simulink model "FixedWing_Dynamic_Model_SIL_simulink_PX4_H200"  (R2023a)
settings: Solver=ode4  StartTime=0.0  StopTime=130  FixedStep=0.004  RelTol=1e-3
model workspace (MAT data in the model file):
  sample_time = 0.004
values from neighbouring files (symbols this model uses):
  ref_height = 171    [InitSimulinkPlantVars.m]
  ref_lat = 39.49738807491014    (= 39.4973880749)    [InitSimulinkPlantVars.m]
  ref_lon = -0.6268122488722822    (= -0.626812248872)    [InitSimulinkPlantVars.m]
undefined symbols (not defined in the file or in its folder): DiscIntNeverNeededParam, Earth, env, frecuency, g, LC, mission, nwap, pitch_D, pitch_ff, pitch_I, pitch_P, poswp, roll_D, roll_ff, roll_I, roll_P, tc_pitch, tc_roll, TEBCL, TECL, TECS, uavData, V_cruise, WGS84, yaw_D, yaw_ff, yaw_I, yaw_P
libraries: aerolibactuator x5, aerolibasang x4, slpidlib x3, uavalgslib x2, aerolibatmos2 x2, shared6dof x1, aerolibtransform2 x1, simulink_extras x1
(part 2 of 3)

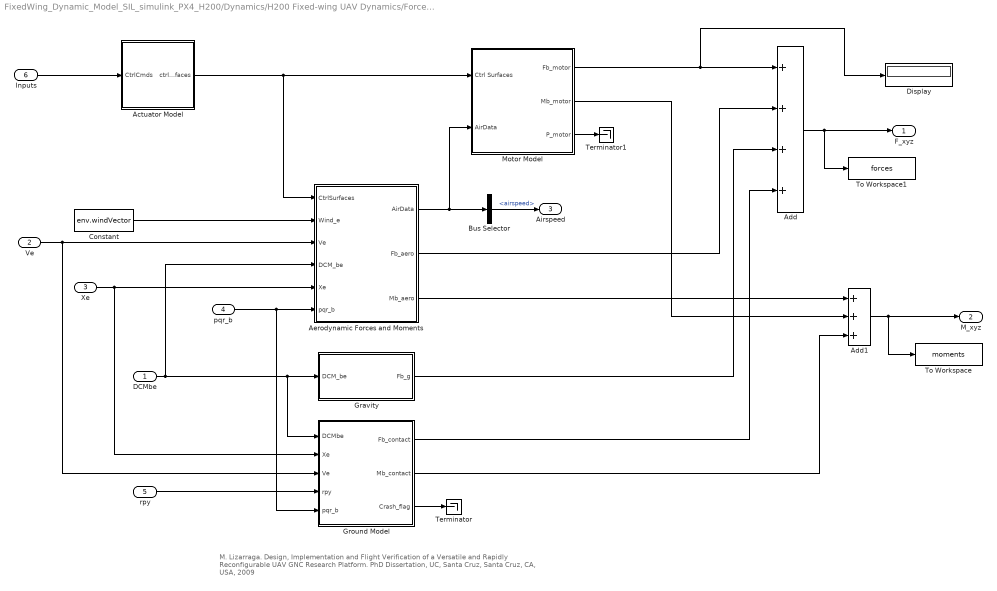
== system FixedWing_Dynamic_Model_SIL_simulink_PX4_H200/Dynamics/H200 Fixed-wing UAV Dynamics/Force and Moment Calculation ==
  note: M. Lizarraga. Design, Implementation and Flight Verification of a Versatile and Rapidly Reconfigurable UAV GNC Research Platform. PhD Dissertation, UC, Santa Cruz, Santa Cruz, CA, USA, 2009
  DCMbe : Inport
  Ve : Inport  Port=2
  Xe : Inport  Port=3
  pqr_b : Inport  Port=4
  rpy : Inport  Port=5
  Inputs : Inport  Port=6
  Actuator Model : Subsystem
  Add : Sum  Inputs=4
  Add1 : Sum  Inputs=+++
  Aerodynamic Forces and Moments : Subsystem
  Bus Selector : BusSelector  OutputSignals=airspeed
  Constant : Constant  Value=env.windVector
  Display : Display
  Gravity : Subsystem
  Ground Model : Subsystem
  Motor Model : Subsystem
  Terminator : Terminator
  Terminator1 : Terminator
  To Workspace : ToWorkspace  VariableName=moments  SaveFormat=Timeseries  SampleTime=-1
  To Workspace1 : ToWorkspace  VariableName=forces  SaveFormat=Timeseries  SampleTime=-1
  F_xyz : Outport
  M_xyz : Outport  Port=2
  Airspeed : Outport  Port=3
  wires:
  Add/1 -> To Workspace1/1, F_xyz/1
  DCMbe/1 -> Ground Model/1(DCMbe), Gravity/1(DCM_be), Aerodynamic Forces and Moments/4(DCM_be)
  pqr_b/1 -> Aerodynamic Forces and Moments/6(pqr_b), Ground Model/5(pqr_b)
  Actuator Model/1(ctrlSurfaces) -> Aerodynamic Forces and Moments/1(CtrlSurfaces), Motor Model/1(Ctrl Surfaces)
  Aerodynamic Forces and Moments/1(AirData) -> Motor Model/2(AirData), Bus Selector/1
  Ground Model/1(Fb_contact) -> Add/4
  Gravity/1(Fb_g) -> Add/3
  Motor Model/1(Fb_motor) -> Display/1, Add/1
  Ve/1 -> Aerodynamic Forces and Moments/3(Ve), Ground Model/3(Ve)
  Ground Model/3(Crash_flag) -> Terminator/1
  Aerodynamic Forces and Moments/2(Fb_aero) -> Add/2
  Aerodynamic Forces and Moments/3(Mb_aero) -> Add1/1
  Xe/1 -> Aerodynamic Forces and Moments/5(Xe), Ground Model/2(Xe)
  Constant/1 -> Aerodynamic Forces and Moments/2(Wind_e)
  Inputs/1 -> Actuator Model/1(CtrlCmds)
  Bus Selector/1 -> Airspeed/1  "<airspeed>"
  rpy/1 -> Ground Model/4(rpy)
  Add1/1 -> M_xyz/1, To Workspace/1
  Ground Model/2(Mb_contact) -> Add1/3
  Motor Model/2(Mb_motor) -> Add1/2
  Motor Model/3(P_motor) -> Terminator1/1

== system FixedWing_Dynamic_Model_SIL_simulink_PX4_H200/Controllers/Total Energy control system/Total energy balance control loop/ B SP dot ==
  h : Inport  SampleTime=frecuency
  V_TAS : Inport  Port=2  SampleTime=frecuency
  V_TAS_sp : Inport  Port=3  SampleTime=frecuency
  h_sp : Inport  Port=4  SampleTime=frecuency
  h_rate_sp : Inport  Port=5  SampleTime=frecuency
  weight_ske : Inport  Port=6  SampleTime=frecuency
  weight_spe : Inport  Port=7  SampleTime=frecuency
  Add : Sum  Inputs=-+
  Add1 : Sum  Inputs=-+
  Add2 : Sum  Inputs=-+
  Add3 : Sum
  Constant : Constant  Value=TECL.V_error_gain  SampleTime=frecuency
  Constant1 : Constant  Value=TECL.h_error_gain  SampleTime=frecuency
  Constant2 : Constant  Value=TECL.h_ff_gain  SampleTime=frecuency
  Constant3 : Constant  Value=g  SampleTime=frecuency
  Product1 : Product
  Product2 : Product  Inputs=3
  Product3 : Product
  Product4 : Product
  Product5 : Product  Inputs=3
  Bdot SP : Outport  SampleTime=frecuency
  wires:
  V_TAS_sp/1 -> Add1/2
  Product1/1 -> Product2/2
  Product2/1 -> Add/1  "kinetic"
  h_sp/1 -> Add2/2
  h/1 -> Add2/1
  Add2/1 -> Product4/2
  Constant1/1 -> Product4/1
  Product4/1 -> Add3/1
  Constant2/1 -> Product3/1
  Product3/1 -> Add3/2
  Add3/1 -> Product5/2
  Constant3/1 -> Product5/1
  Product5/1 -> Add/2  "potential"
  Add/1 -> Bdot SP/1
  h_rate_sp/1 -> Product3/2
  weight_ske/1 -> Product2/3
  weight_spe/1 -> Product5/3
  V_TAS/1 -> Add1/1, Product2/1
  Add1/1 -> Product1/1
  Constant/1 -> Product1/2

== system FixedWing_Dynamic_Model_SIL_simulink_PX4_H200/Controllers/Total Energy control system/Total energy balance control loop/Bdot ==
  V_TAS : Inport  SampleTime=frecuency
  V_rate : Inport  Port=2  SampleTime=frecuency
  h_rate : Inport  Port=3  SampleTime=frecuency
  weight_ske : Inport  Port=4  SampleTime=frecuency
  weight_spe : Inport  Port=5  SampleTime=frecuency
  Add : Sum  Inputs=-+
  Constant : Constant  Value=g  SampleTime=frecuency
  Product : Product  Inputs=3
  Product1 : Product  Inputs=3
  Bdot : Outport  SampleTime=frecuency
  wires:
  V_rate/1 -> Product/2
  Constant/1 -> Product1/3
  h_rate/1 -> Product1/2
  Product/1 -> Add/1  "kinetic"
  Product1/1 -> Add/2  "potential"
  Add/1 -> Bdot/1
  weight_ske/1 -> Product/3
  weight_spe/1 -> Product1/1
  V_TAS/1 -> Product/1

== system FixedWing_Dynamic_Model_SIL_simulink_PX4_H200/Controllers/Total Energy control system/Total energy balance control loop/pitchdotsp - pitchFF ==
  Bdot SP : Inport  SampleTime=frecuency
  Gain : Gain  Gain=TEBCL.rate_ff
  pitch_FF : Outport  SampleTime=frecuency
  wires:
  Bdot SP/1 -> Gain/1
  Gain/1 -> pitch_FF/1

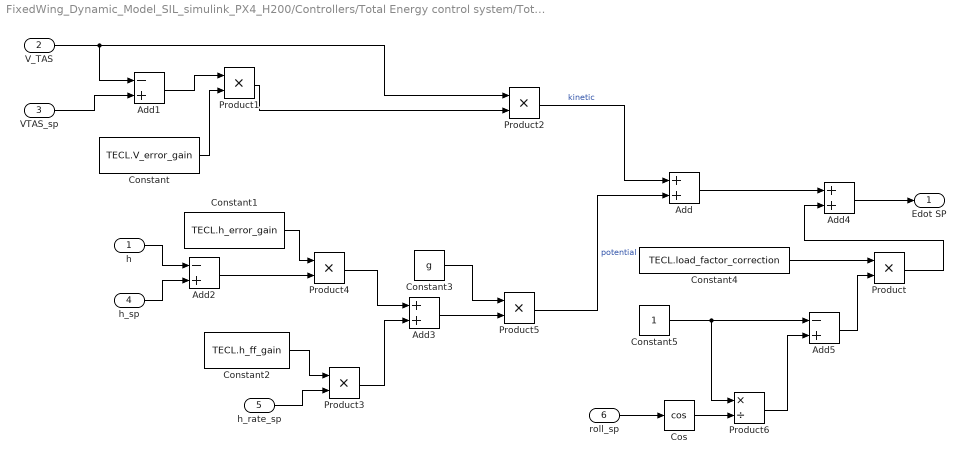
== system FixedWing_Dynamic_Model_SIL_simulink_PX4_H200/Controllers/Total Energy control system/Total energy control loop/E SP dot ==
  h : Inport  SampleTime=frecuency
  V_TAS : Inport  Port=2  SampleTime=frecuency
  VTAS_sp : Inport  Port=3  SampleTime=frecuency
  h_sp : Inport  Port=4  SampleTime=frecuency
  h_rate_sp : Inport  Port=5  SampleTime=frecuency
  roll_sp : Inport  Port=6  SampleTime=frecuency
  Add : Sum
  Add1 : Sum  Inputs=-+
  Add2 : Sum  Inputs=-+
  Add3 : Sum
  Add4 : Sum
  Add5 : Sum  Inputs=-+
  Constant : Constant  Value=TECL.V_error_gain  SampleTime=frecuency
  Constant1 : Constant  Value=TECL.h_error_gain  SampleTime=frecuency
  Constant2 : Constant  Value=TECL.h_ff_gain  SampleTime=frecuency
  Constant3 : Constant  Value=g
  Constant4 : Constant  Value=TECL.load_factor_correction  SampleTime=frecuency
  Constant5 : Constant
  Cos : Trigonometry  Operator=cos
  Product{,1..5} (6 alike) : Product
  Product6 : Product  Inputs=*/
  Edot SP : Outport  SampleTime=frecuency
  wires:
  VTAS_sp/1 -> Add1/2
  Product2/1 -> Add/1  "kinetic"
  h_sp/1 -> Add2/2
  h/1 -> Add2/1
  Add2/1 -> Product4/2
  Constant1/1 -> Product4/1
  Product4/1 -> Add3/1
  Constant2/1 -> Product3/1
  Product3/1 -> Add3/2
  Add3/1 -> Product5/2
  Constant3/1 -> Product5/1
  Product5/1 -> Add/2  "potential"
  h_rate_sp/1 -> Product3/2
  Add/1 -> Add4/1
  Add4/1 -> Edot SP/1
  Constant4/1 -> Product/1
  Product/1 -> Add4/2
  Constant5/1 -> Add5/1, Product6/1
  Add5/1 -> Product/2
  roll_sp/1 -> Cos/1
  Cos/1 -> Product6/2
  Product6/1 -> Add5/2
  Constant/1 -> Product1/2
  Add1/1 -> Product1/1
  Product1/1 -> Product2/2
  V_TAS/1 -> Product2/1, Add1/1

== system FixedWing_Dynamic_Model_SIL_simulink_PX4_H200/Controllers/Total Energy control system/Total energy control loop/Edot ==
  V_TAS : Inport  SampleTime=frecuency
  V_rate : Inport  Port=2  SampleTime=frecuency
  h_rate : Inport  Port=3  SampleTime=frecuency
  Add : Sum
  Constant : Constant  Value=g  SampleTime=frecuency
  Product : Product
  Product1 : Product
  Edot : Outport  SampleTime=frecuency
  wires:
  V_TAS/1 -> Product/1
  V_rate/1 -> Product/2
  Constant/1 -> Product1/2
  h_rate/1 -> Product1/1
  Product/1 -> Add/1  "kinetic"
  Product1/1 -> Add/2  "potential"
  Add/1 -> Edot/1

== system FixedWing_Dynamic_Model_SIL_simulink_PX4_H200/Controllers/Total Energy control system/Total energy control loop/Subsystem ==
  ratio_undersped : Inport  SampleTime=frecuency
  T_sp : Inport  Port=2  SampleTime=frecuency
  Tmax : Inport  Port=3  SampleTime=frecuency
  Add : Sum  Inputs=+-
  Add1 : Sum
  Constant : Constant  SampleTime=frecuency
  Product : Product
  Product1 : Product
  throttle_setpoint : Outport  SampleTime=frecuency
  wires:
  ratio_undersped/1 -> Product/1, Add/2
  Tmax/1 -> Product/2
  Constant/1 -> Add/1
  T_sp/1 -> Product1/1
  Add/1 -> Product1/2
  Product1/1 -> Add1/1
  Product/1 -> Add1/2
  Add1/1 -> throttle_setpoint/1

== system FixedWing_Dynamic_Model_SIL_simulink_PX4_H200/Controllers/Total Energy control system/Total energy control loop/Subsystem1 ==
  throttle_integ_input : Inport  SampleTime=frecuency
  ste_rate_to_throttle : Inport  Port=2  SampleTime=frecuency
  ratio_undersped : Inport  Port=3  SampleTime=frecuency
  Add : Sum  Inputs=-+
  Constant : Constant  SampleTime=frecuency
  Product : Product  Inputs=3
  throttle_integ : Outport  SampleTime=frecuency
  wires:
  ratio_undersped/1 -> Add/1
  Constant/1 -> Add/2
  throttle_integ_input/1 -> Product/1
  ste_rate_to_throttle/1 -> Product/2
  Add/1 -> Product/3
  Product/1 -> throttle_integ/1

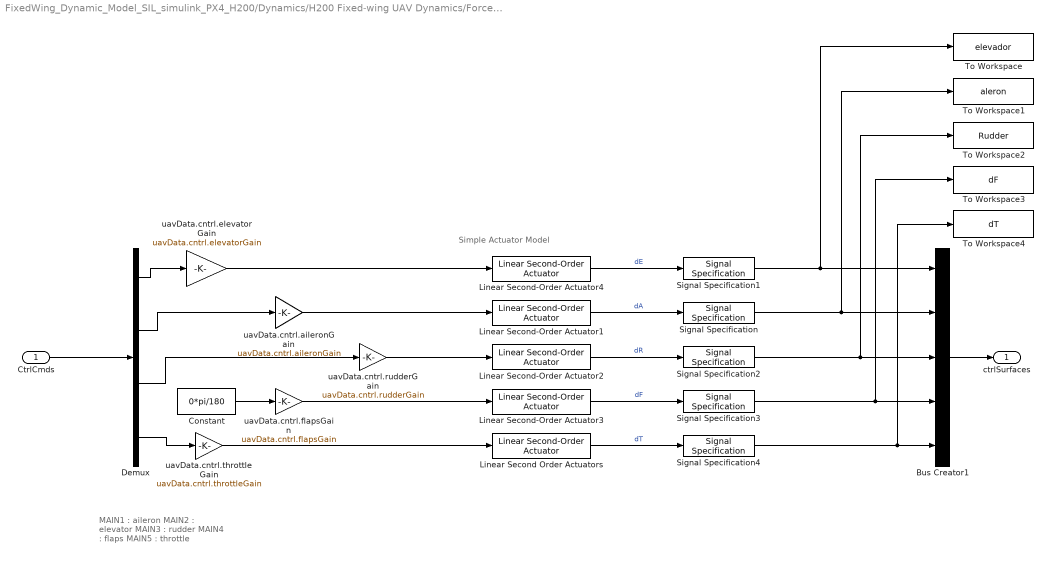
== system FixedWing_Dynamic_Model_SIL_simulink_PX4_H200/Dynamics/H200 Fixed-wing UAV Dynamics/Force and Moment Calculation/Actuator Model ==
  note: Simple Actuator Model
  note: MAIN1 : aileron
      | MAIN2 : elevator
      | MAIN3 : rudder
      | MAIN4 : flaps
      | MAIN5 : throttle
  CtrlCmds : Inport
  Bus Creator1 : BusCreator  Inputs=5
  Constant : Constant  Value=0*pi/180
  Demux : Demux
  Linear Second Order Actuators : aerolibactuator/Linear Second-Order Actuator  wn_fin=uavData.cntrl.naturalFreq  z_fin=uavData.cntrl.dampingRatio  fin_act_0=uavData.cntrl.initPos  fin_act_vel=uavData.cntrl.initVel
      settings: AttributesFormatString=|
      | Nat Freq => %<wn_fin>
      | Damping => %<z_fin>
  Linear Second-Order Actuator{1..4} (4 alike) : aerolibactuator/Linear Second-Order Actuator  wn_fin=uavData.cntrl.naturalFreq  z_fin=uavData.cntrl.dampingRatio  fin_act_0=uavData.cntrl.initPos  fin_act_vel=uavData.cntrl.initVel
  Signal Specification{,1..3} (4 alike) : SignalSpecification  Unit=rad
  Signal Specification4 : SignalSpecification  Unit=%
  To Workspace : ToWorkspace  VariableName=elevador  SaveFormat=Timeseries  SampleTime=-1
  To Workspace1 : ToWorkspace  VariableName=aleron  SaveFormat=Timeseries  SampleTime=-1
  To Workspace2 : ToWorkspace  VariableName=Rudder  SaveFormat=Timeseries  SampleTime=-1
  To Workspace3 : ToWorkspace  VariableName=dF  SaveFormat=Timeseries  SampleTime=-1
  To Workspace4 : ToWorkspace  VariableName=dT  SaveFormat=Timeseries  SampleTime=-1
  uavData.cntrl.aileronGain : Gain  Gain=uavData.cntrl.aileronGain
  uavData.cntrl.elevatorGain : Gain  Gain=uavData.cntrl.elevatorGain
  uavData.cntrl.flapsGain : Gain  Gain=uavData.cntrl.flapsGain
  uavData.cntrl.rudderGain : Gain  Gain=uavData.cntrl.rudderGain
  uavData.cntrl.throttleGain : Gain  Gain=uavData.cntrl.throttleGain
  ctrlSurfaces : Outport  VectorParamsAs1DForOutWhenUnconnected=off
  wires:
  uavData.cntrl.throttleGain/1 -> Linear Second Order Actuators/1
  Bus Creator1/1 -> ctrlSurfaces/1
  Linear Second-Order Actuator4/1 -> Signal Specification1/1  "dE"
  Linear Second-Order Actuator1/1 -> Signal Specification/1  "dA"
  Linear Second-Order Actuator2/1 -> Signal Specification2/1  "dR"
  Linear Second-Order Actuator3/1 -> Signal Specification3/1  "dF"
  Linear Second Order Actuators/1 -> Signal Specification4/1  "dT"
  CtrlCmds/1 -> Demux/1
  Signal Specification1/1 -> To Workspace/1, Bus Creator1/1
  Signal Specification/1 -> To Workspace1/1, Bus Creator1/2
  Signal Specification2/1 -> To Workspace2/1, Bus Creator1/3
  Signal Specification3/1 -> To Workspace3/1, Bus Creator1/4
  Signal Specification4/1 -> Bus Creator1/5, To Workspace4/1
  Demux/3 -> uavData.cntrl.rudderGain/1
  Demux/1 -> uavData.cntrl.elevatorGain/1
  Demux/2 -> uavData.cntrl.aileronGain/1
  uavData.cntrl.elevatorGain/1 -> Linear Second-Order Actuator4/1
  uavData.cntrl.rudderGain/1 -> Linear Second-Order Actuator2/1
  uavData.cntrl.aileronGain/1 -> Linear Second-Order Actuator1/1
  uavData.cntrl.flapsGain/1 -> Linear Second-Order Actuator3/1
  Demux/4 -> uavData.cntrl.throttleGain/1
  Constant/1 -> uavData.cntrl.flapsGain/1

== system FixedWing_Dynamic_Model_SIL_simulink_PX4_H200/Dynamics/H200 Fixed-wing UAV Dynamics/Force and Moment Calculation/Aerodynamic Forces and Moments ==
  CtrlSurfaces : Inport
  Wind_e : Inport  Port=2
  Ve : Inport  Port=3
  DCM_be : Inport  Port=4
  Xe : Inport  Port=5
  pqr_b : Inport  Port=6
  Compute Air Data : Subsystem  TreatAsAtomicUnit=on  VariantControl=use_aerospace_blocks == 1
  Compute Body Frame Forces and Moments : Subsystem
  Compute Rho : Subsystem
  Rotate Vw : Subsystem
  Vair : Sum  Inputs=+-  InputSameDT=on  SaturateOnIntegerOverflow=on  OutDataTypeStr=Inherit: Same as first input
  AirData : Outport  VectorParamsAs1DForOutWhenUnconnected=off
  Fb_aero : Outport  Port=2
  Mb_aero : Outport  Port=3
  wires:
  Ve/1 -> Vair/1
  Compute Body Frame Forces and Moments/1(F_b) -> Fb_aero/1
  Wind_e/1 -> Vair/2
  CtrlSurfaces/1 -> Compute Body Frame Forces and Moments/2(CtrlSurfaces)
  Compute Air Data/1(AirData) -> Compute Body Frame Forces and Moments/1(AirData), AirData/1
  Compute Body Frame Forces and Moments/2(M_b) -> Mb_aero/1
  Rotate Vw/1(Vb) -> Compute Air Data/1(Vb)
  Compute Rho/1(Rho) -> Compute Air Data/2(Rho)
  Vair/1 -> Rotate Vw/1(Vw)
  pqr_b/1 -> Compute Body Frame Forces and Moments/3(p,q,r)
  DCM_be/1 -> Rotate Vw/2(DCM_be)
  Xe/1 -> Compute Rho/1(Xe)

== system FixedWing_Dynamic_Model_SIL_simulink_PX4_H200/Dynamics/H200 Fixed-wing UAV Dynamics/Force and Moment Calculation/Gravity ==
  DCM_be : Inport
  Constant : Constant  Value=[0 0 env.ISA_g]'
  Gain : Gain  Gain=uavData.geometry.m
  Matrix Multiply : Product  Multiplication=Matrix(*)
  Fb_g : Outport
  wires:
  Matrix Multiply/1 -> Gain/1
  Constant/1 -> Matrix Multiply/2
  DCM_be/1 -> Matrix Multiply/1
  Gain/1 -> Fb_g/1

== system FixedWing_Dynamic_Model_SIL_simulink_PX4_H200/Dynamics/H200 Fixed-wing UAV Dynamics/Force and Moment Calculation/Ground Model ==
  note: Body is assumed to be a rigid point mass on ground for contact force calculations.
      |
      | Normal force is modelled as a spring mass damper.
      |
      | Friction is modelled using Soft Coulomb model.
  DCMbe : Inport
  Xe : Inport  Port=2
  Ve : Inport  Port=3
  rpy : Inport  Port=4
  pqr_b : Inport  Port=5
  Constant : Constant  Value=[0 0 0]
  Crash Detector : Subsystem
  Friction Force : Subsystem
  Matrix Multiply : Product  Multiplication=Matrix(*)
  Mux1 : Mux  Inputs=2
  Normal Force : Subsystem
  Selector : Selector  InputPortWidth=3  IndexOptions=Index vector (dialog)  Indices=[3]  OutputSizes=1
  Selector1 : Selector  InputPortWidth=3  IndexOptions=Index vector (dialog)  Indices=[3]  OutputSizes=1
  Selector2 : Selector  InputPortWidth=3  IndexOptions=Index vector (dialog)  Indices=[1,2]  OutputSizes=1
  Terminator : Terminator
  Terminator1 : Terminator
  Unary Minus1 : UnaryMinus
  Fb_contact : Outport
  Mb_contact : Outport  Port=2
  Crash_flag : Outport  Port=3
  wires:
  Crash Detector/1(crashFlag) -> Crash_flag/1
  Xe/1 -> Selector/1
  Ve/1 -> Selector2/1, Selector1/1
  Selector1/1 -> Normal Force/1(Vz)
  Selector/1 -> Normal Force/2(Z)
  DCMbe/1 -> Matrix Multiply/1
  Matrix Multiply/1 -> Fb_contact/1
  Normal Force/1(Normal) -> Friction Force/2(Fn), Unary Minus1/1
  Mux1/1 -> Matrix Multiply/2, Crash Detector/1(F)
  Unary Minus1/1 -> Mux1/2
  Selector2/1 -> Friction Force/1(V)
  Friction Force/1(Friction) -> Mux1/1
  pqr_b/1 -> Terminator/1
  rpy/1 -> Terminator1/1
  Constant/1 -> Mb_contact/1

== system FixedWing_Dynamic_Model_SIL_simulink_PX4_H200/Dynamics/H200 Fixed-wing UAV Dynamics/Force and Moment Calculation/Motor Model ==
  Ctrl Surfaces : Inport
  AirData : Inport  Port=2
  Bus Selector : BusSelector  OutputSignals=dT
  Constant2 : Constant  Value=uavData.geometry.LProp
  Engine Model : Subsystem
  Gain1 : Gain  Gain=-1
  Product1 : Product  Inputs=**
  Fb_motor : Outport  VectorParamsAs1DForOutWhenUnconnected=off
  Mb_motor : Outport  Port=2  VectorParamsAs1DForOutWhenUnconnected=off
  P_motor : Outport  Port=3  VectorParamsAs1DForOutWhenUnconnected=off
  wires:
  Ctrl Surfaces/1 -> Bus Selector/1
  Bus Selector/1 -> Engine Model/1(dt)  "<dT>"
  Engine Model/1(Thrust_b) -> Fb_motor/1, Product1/1
  Constant2/1 -> Product1/2
  Product1/1 -> Gain1/1
  Gain1/1 -> Mb_motor/1
  AirData/1 -> Engine Model/2(AirData)
  Engine Model/2(Power) -> P_motor/1

== system FixedWing_Dynamic_Model_SIL_simulink_PX4_H200/Dynamics/H200 Fixed-wing UAV Dynamics/Force and Moment Calculation/Aerodynamic Forces and Moments/Compute Air Data ==
  Vb : Inport  PortDimensions=3
  Rho : Inport  Port=2
  Bus Creator : BusCreator  Inputs=4
  Demux : Demux  Outputs=3
  Dynamic Pressure : aerolibasang/Dynamic Pressure
  Subsystem : Subsystem
  AirData : Outport  VectorParamsAs1DForOutWhenUnconnected=off
  wires:
  Bus Creator/1 -> AirData/1
  Rho/1 -> Dynamic Pressure/2
  Dynamic Pressure/1 -> Bus Creator/4  "q"
  Vb/1 -> Subsystem/1(Vb), Dynamic Pressure/1
  Subsystem/1(airData) -> Demux/1
  Demux/1 -> Bus Creator/1  "alpha"
  Demux/2 -> Bus Creator/2  "beta"
  Demux/3 -> Bus Creator/3  "airspeed"

== system FixedWing_Dynamic_Model_SIL_simulink_PX4_H200/Dynamics/H200 Fixed-wing UAV Dynamics/Force and Moment Calculation/Aerodynamic Forces and Moments/Compute Body Frame Forces and Moments ==
  AirData : Inport
  CtrlSurfaces : Inport  Port=2
  p,q,r : Inport  Port=3
  Bus Selector : BusSelector  OutputSignals=alpha,beta
  Mux : Mux  Inputs=2
  Rotate FM to body frame : Subsystem
  Wind frame F& M : Subsystem
  F_b : Outport  Unit=kg*m/s^2  VectorParamsAs1DForOutWhenUnconnected=off
  M_b : Outport  Port=2  Unit=N*m  VectorParamsAs1DForOutWhenUnconnected=off
  wires:
  Mux/1 -> Rotate FM to body frame/2(alpha_beta)
  Bus Selector/2 -> Mux/2  "<beta>"
  Bus Selector/1 -> Mux/1  "<alpha>"
  Wind frame F& M/1(FM_w) -> Rotate FM to body frame/1(FM_w)  "FM_W"
  p,q,r/1 -> Wind frame F& M/3(p,q,r)
  Rotate FM to body frame/2(M_b) -> M_b/1
  Rotate FM to body frame/1(F_b) -> F_b/1
  CtrlSurfaces/1 -> Wind frame F& M/2(CtrlSurfaces)
  AirData/1 -> Wind frame F& M/1(Airdata), Bus Selector/1

== system FixedWing_Dynamic_Model_SIL_simulink_PX4_H200/Dynamics/H200 Fixed-wing UAV Dynamics/Force and Moment Calculation/Aerodynamic Forces and Moments/Compute Rho ==
  Xe : Inport
  Gain : Gain  Gain=-1
      settings: AttributesFormatString=Z to Alt
  Get Z : Selector  InputPortWidth=3  IndexOptions=Index vector (dialog)  Indices=[3]  OutputSizes=[(-2)]
  ISA Atmosphere Model1 : aerolibatmos2/ISA Atmosphere Model  custom=on  g=env.ISA_g  gamma=1.4  R=env.ISA_R  L=env.ISA_lapse  h_trop=11000  h_strat=20000  rho0=env.ISA_rho0  P0=env.ISA_P0  T0=env.ISA_T0  h0=0
  Terminator : Terminator
  Terminator1 : Terminator
  Terminator2 : Terminator
  Transfer Fcn : TransferFcn  Denominator=[.01 1]
  Rho : Outport  VectorParamsAs1DForOutWhenUnconnected=off
  wires:
  ISA Atmosphere Model1/2 -> Terminator1/1
  ISA Atmosphere Model1/1 -> Terminator/1  "OAT"
  Gain/1 -> ISA Atmosphere Model1/1
  Get Z/1 -> Transfer Fcn/1
  Transfer Fcn/1 -> Gain/1
  ISA Atmosphere Model1/3 -> Terminator2/1  "static"
  Xe/1 -> Get Z/1
  ISA Atmosphere Model1/4 -> Rho/1

== system FixedWing_Dynamic_Model_SIL_simulink_PX4_H200/Dynamics/H200 Fixed-wing UAV Dynamics/Force and Moment Calculation/Aerodynamic Forces and Moments/Rotate Vw ==
  Vw : Inport
  DCM_be : Inport  Port=2
  RL2B * Vw : Product  Multiplication=Matrix(*)  InputSameDT=on  SaturateOnIntegerOverflow=on  OutDataTypeStr=Inherit: Same as first input
  Vb : Outport  Unit=m/s  VectorParamsAs1DForOutWhenUnconnected=off
  wires:
  RL2B * Vw/1 -> Vb/1
  Vw/1 -> RL2B * Vw/2
  DCM_be/1 -> RL2B * Vw/1

== system FixedWing_Dynamic_Model_SIL_simulink_PX4_H200/Dynamics/H200 Fixed-wing UAV Dynamics/Force and Moment Calculation/Ground Model/Crash Detector ==
  F : Inport
  Constant : Constant  Value=true
  Constant1 : Constant  Value=false
  Gain : Gain  Gain=1/(env.ISA_g*uavData.geometry.m)
  Switch : Switch  Criteria=u2 > Threshold  Threshold=uavData.contact.gLimit  SaturateOnIntegerOverflow=off  InputSameDT=off
  norm1 : Subsystem
  crashFlag : Outport
  wires:
  F/1 -> norm1/1(F)
  norm1/1(Out1) -> Gain/1
  Switch/1 -> crashFlag/1
  Constant/1 -> Switch/1
  Constant1/1 -> Switch/3
  Gain/1 -> Switch/2

== system FixedWing_Dynamic_Model_SIL_simulink_PX4_H200/Dynamics/H200 Fixed-wing UAV Dynamics/Force and Moment Calculation/Ground Model/Friction Force ==
  V : Inport
  Fn : Inport  Port=2
  Product : Product
  Soft Coulomb Friction : Subsystem
  Unary Minus : UnaryMinus
  Friction : Outport
  wires:
  Fn/1 -> Product/2
  Soft Coulomb Friction/1(Out1) -> Product/1
  Product/1 -> Unary Minus/1
  Unary Minus/1 -> Friction/1
  V/1 -> Soft Coulomb Friction/1(V)

== system FixedWing_Dynamic_Model_SIL_simulink_PX4_H200/Dynamics/H200 Fixed-wing UAV Dynamics/Force and Moment Calculation/Ground Model/Normal Force ==
  Vz : Inport
  Z : Inport  Port=2
  Add : Sum
  Constant : Constant  Value=0
  Damper : Gain  Gain=-uavData.contact.damper
  Saturation : Saturate  UpperLimit=inf  LowerLimit=0
  Spring Kp : Gain  Gain=-uavData.contact.spring
  Switch : Switch  Criteria=u2 > Threshold  SaturateOnIntegerOverflow=off  InputSameDT=off
  Unary Minus : UnaryMinus
  Unary Minus1 : UnaryMinus
  Normal : Outport
  wires:
  Constant/1 -> Switch/1
  Z/1 -> Unary Minus/1
  Switch/1 -> Saturation/1
  Damper/1 -> Add/2
  Add/1 -> Switch/3
  Spring Kp/1 -> Add/1
  Vz/1 -> Unary Minus1/1
  Saturation/1 -> Normal/1
  Unary Minus/1 -> Spring Kp/1, Switch/2
  Unary Minus1/1 -> Damper/1

== system FixedWing_Dynamic_Model_SIL_simulink_PX4_H200/Dynamics/H200 Fixed-wing UAV Dynamics/Force and Moment Calculation/Motor Model/Engine Model ==
  dt : Inport
  AirData : Inport  Port=2
  Constant4 : Constant  Value=0
      settings: AttributesFormatString=%<Value>
  Mux1 : Mux  Inputs=3
  Power Model : Subsystem
  Thurst Model : Subsystem
  To Workspace1 : ToWorkspace  VariableName=thrustMotor  SaveFormat=Timeseries  SampleTime=-1
  To Workspace2 : ToWorkspace  VariableName=powerMotor  SaveFormat=Timeseries  SampleTime=-1
  Thrust_b : Outport  Unit=kg*m/s^2  VectorParamsAs1DForOutWhenUnconnected=off
  Power : Outport  Port=2  Unit=kg*m/s^2  VectorParamsAs1DForOutWhenUnconnected=off
  wires:
  Constant4/1 -> Mux1/2, Mux1/3
  Mux1/1 -> Thrust_b/1
  dt/1 -> Power Model/1(dt), Thurst Model/1(dt)
  Thurst Model/1(T_Total) -> Mux1/1, To Workspace1/1
  AirData/1 -> Thurst Model/2(AirData), Power Model/2(AirData)
  Power Model/1(P_Total) -> To Workspace2/1, Power/1

== system FixedWing_Dynamic_Model_SIL_simulink_PX4_H200/Dynamics/H200 Fixed-wing UAV Dynamics/Force and Moment Calculation/Aerodynamic Forces and Moments/Compute Air Data/Subsystem ==
  note: Avoid singularity at low speeds
  Vb : Inport
  "Incidence, Sideslip, & Airspeed" : aerolibasang/Incidence, Sideslip, & Airspeed
  Mux : Mux  Inputs=3
  Mux1 : Mux  Inputs=3
  Switch : Switch  Criteria=u2 > Threshold  Threshold=0.1  SaturateOnIntegerOverflow=off  InputSameDT=off
  alpha : Constant  Value=0
  beta : Constant  Value=0
  norm : Subsystem
  airData : Outport
  wires:
  "Incidence, Sideslip, & Airspeed"/1 -> Mux/1  "alpha"
  "Incidence, Sideslip, & Airspeed"/3 -> Mux/3  "airspeed"
  Vb/1 -> norm/1(In1), "Incidence, Sideslip, & Airspeed"/1
  norm/1(Out1) -> Switch/2, Mux1/3
  "Incidence, Sideslip, & Airspeed"/2 -> Mux/2  "beta"
  Switch/1 -> airData/1
  Mux/1 -> Switch/1
  alpha/1 -> Mux1/1
  beta/1 -> Mux1/2
  Mux1/1 -> Switch/3

== system FixedWing_Dynamic_Model_SIL_simulink_PX4_H200/Dynamics/H200 Fixed-wing UAV Dynamics/Force and Moment Calculation/Aerodynamic Forces and Moments/Compute Body Frame Forces and Moments/Rotate FM to body frame ==
  FM_w : Inport
  alpha_beta : Inport  Port=2
  Forces : Selector  InputPortWidth=6  IndexOptions=Index vector (dialog)  Indices=[1 2 3]  OutputSizes=[(-2)]
  Moments : Selector  InputPortWidth=6  IndexOptions=Index vector (dialog)  Indices=[4 5 6]  OutputSizes=[(-2)]
  Rotate Forces : Subsystem
  Rotate Moments : Subsystem
  F_b : Outport  VectorParamsAs1DForOutWhenUnconnected=off
  M_b : Outport  Port=2  VectorParamsAs1DForOutWhenUnconnected=off
  wires:
  alpha_beta/1 -> Rotate Forces/2(alpha_beta), Rotate Moments/1(alpha_beta)
  Moments/1 -> Rotate Moments/2(M_w)
  FM_w/1 -> Forces/1, Moments/1
  Forces/1 -> Rotate Forces/1(F_w)
  Rotate Moments/1(M_b) -> M_b/1
  Rotate Forces/1(F_b) -> F_b/1

== system FixedWing_Dynamic_Model_SIL_simulink_PX4_H200/Dynamics/H200 Fixed-wing UAV Dynamics/Force and Moment Calculation/Aerodynamic Forces and Moments/Compute Body Frame Forces and Moments/Wind frame F& M ==
  Airdata : Inport
  CtrlSurfaces : Inport  Port=2
  p,q,r : Inport  Port=3
  Bus Creator1 : BusCreator  Inputs=2
  Bus Selector1 : BusSelector  OutputSignals=dA,dR
  Bus Selector2 : BusSelector  OutputSignals=dE,dF
  Bus Selector6 : BusSelector  OutputSignals=beta,airspeed
  Bus Selector7 : BusSelector  OutputSignals=alpha,airspeed
  Get Forces and Moments : Subsystem
  Lateral Channel : Subsystem
  Longitudinal Channel : Subsystem
  To Workspace : ToWorkspace  VariableName=alpha  SaveFormat=Timeseries  SampleTime=-1
  FM_w : Outport  PortDimensions=6  VectorParamsAs1DForOutWhenUnconnected=off
  wires:
  Get Forces and Moments/1(FM_w) -> FM_w/1
  Bus Creator1/1 -> Get Forces and Moments/2(AeroCoeffs)
  Bus Selector7/2 -> Longitudinal Channel/2(Airpseed)  "<airspeed>"
  Bus Selector7/1 -> To Workspace/1, Longitudinal Channel/1(alpha)  "<alpha>"
  Bus Selector6/2 -> Lateral Channel/3(Airspeed)  "<airspeed>"
  Bus Selector6/1 -> Lateral Channel/1(beta)  "<beta>"
  Airdata/1 -> Bus Selector6/1, Bus Selector7/1, Get Forces and Moments/1(Airdata)
  Bus Selector2/2 -> Longitudinal Channel/5(dF)  "<dF>"
  Bus Selector2/1 -> Longitudinal Channel/4(dE)  "<dE>"
  Bus Selector1/2 -> Lateral Channel/4(dR)  "<dR>"
  Bus Selector1/1 -> Lateral Channel/5(deltaA)  "<dA>"
  CtrlSurfaces/1 -> Bus Selector1/1, Bus Selector2/1
  p,q,r/1 -> Lateral Channel/2(p,q,r), Longitudinal Channel/3(p,q,r)
  Lateral Channel/1(Lateral) -> Bus Creator1/1
  Longitudinal Channel/1(Longitudinal) -> Bus Creator1/2

== system FixedWing_Dynamic_Model_SIL_simulink_PX4_H200/Dynamics/H200 Fixed-wing UAV Dynamics/Force and Moment Calculation/Ground Model/Crash Detector/norm1 ==
  F : Inport
  Dot Product : DotProduct  OutDataTypeStr=Inherit: Inherit via internal rule
  Sqrt : Sqrt
  Out1 : Outport
  wires:
  Dot Product/1 -> Sqrt/1
  F/1 -> Dot Product/2, Dot Product/1
  Sqrt/1 -> Out1/1

== system FixedWing_Dynamic_Model_SIL_simulink_PX4_H200/Dynamics/H200 Fixed-wing UAV Dynamics/Force and Moment Calculation/Ground Model/Friction Force/Soft Coulomb Friction ==
  note: Pennestrì, E., Rossi, V., Salvini, P. et al. Review and comparison of dry friction force models. Nonlinear Dyn 83, 1785–1801 (2016). https://doi.org/10.1007/s11071-015-2485-3
  V : Inport
  Tanh : Trigonometry  Operator=tanh
  friction coefficient : Gain  Gain=uavData.contact.rollingFriction
  vd : Gain  Gain=1/uavData.contact.vd
  Out1 : Outport
  wires:
  V/1 -> vd/1
  vd/1 -> Tanh/1
  Tanh/1 -> friction coefficient/1
  friction coefficient/1 -> Out1/1

== system FixedWing_Dynamic_Model_SIL_simulink_PX4_H200/Dynamics/H200 Fixed-wing UAV Dynamics/Force and Moment Calculation/Motor Model/Engine Model/Power Model ==
  dt : Inport
  AirData : Inport  Port=2
  Bus Selector : BusSelector  OutputSignals=airspeed,q
  CP Model : Subsystem
  Calculate Rho : Subsystem
  Gain : Gain  Gain=uavData.engine.NMotors
  J model : Subsystem
  N [Hz] model : Subsystem
  Power : Subsystem
  P_Total : Outport  VectorParamsAs1DForOutWhenUnconnected=off
  wires:
  Gain/1 -> P_Total/1
  N [Hz] model/1(n) -> J model/1(n), Power/1(n)
  J model/1(J) -> CP Model/1(J)
  dt/1 -> N [Hz] model/1(deltaP)
  AirData/1 -> Bus Selector/1
  Bus Selector/1 -> J model/2(V), Calculate Rho/1(Airspeed)  "<airspeed>"
  Bus Selector/2 -> Calculate Rho/2(q)  "<q>"
  CP Model/1(CP) -> Power/2(CP)
  Calculate Rho/1(rho) -> Power/3(rho)
  Power/1(P) -> Gain/1

== system FixedWing_Dynamic_Model_SIL_simulink_PX4_H200/Dynamics/H200 Fixed-wing UAV Dynamics/Force and Moment Calculation/Motor Model/Engine Model/Thurst Model ==
  dt : Inport
  AirData : Inport  Port=2
  Bus Selector : BusSelector  OutputSignals=airspeed,q
  CT Model : Subsystem
  Calculate Rho : Subsystem
  Constant : Constant  Value=env.ISA_rho0
  Gain1 : Gain  Gain=uavData.engine.NMotors
  J model : Subsystem
  N [Hz] model : Subsystem
  Thrust Force : Subsystem
  T_Total : Outport  VectorParamsAs1DForOutWhenUnconnected=off
  wires:
  AirData/1 -> Bus Selector/1
  Bus Selector/1 -> J model/2(V), Calculate Rho/1(Airspeed)  "<airspeed>"
  Bus Selector/2 -> Calculate Rho/2(q)  "<q>"
  N [Hz] model/1(n) -> Thrust Force/1(n), J model/1(n)
  CT Model/1(CT) -> Thrust Force/2(CT)
  J model/1(J) -> CT Model/1(J)
  Gain1/1 -> T_Total/1
  dt/1 -> N [Hz] model/1(deltaP)
  Thrust Force/1(T) -> Gain1/1
  Constant/1 -> Thrust Force/3(rho)

== system FixedWing_Dynamic_Model_SIL_simulink_PX4_H200/Dynamics/H200 Fixed-wing UAV Dynamics/Force and Moment Calculation/Aerodynamic Forces and Moments/Compute Air Data/Subsystem/norm ==
  In1 : Inport
  Dot Product : DotProduct  OutDataTypeStr=Inherit: Inherit via internal rule
  Sqrt : Sqrt
  Out1 : Outport
  wires:
  In1/1 -> Dot Product/2, Dot Product/1
  Dot Product/1 -> Sqrt/1
  Sqrt/1 -> Out1/1

== system FixedWing_Dynamic_Model_SIL_simulink_PX4_H200/Dynamics/H200 Fixed-wing UAV Dynamics/Force and Moment Calculation/Aerodynamic Forces and Moments/Compute Body Frame Forces and Moments/Rotate FM to body frame/Rotate Forces ==
  F_w : Inport
  alpha_beta : Inport  Port=2
  Product2 : Product  Multiplication=Matrix(*)  SaturateOnIntegerOverflow=on  OutDataTypeStr=Inherit: Same as first input
  RB2W : Subsystem
  RW2B : Math  Operator=transpose  SignedPower=on
  F_b : Outport  PortDimensions=3  VectorParamsAs1DForOutWhenUnconnected=off
  wires:
  RW2B/1 -> Product2/1
  F_w/1 -> Product2/2
  Product2/1 -> F_b/1
  alpha_beta/1 -> RB2W/1(aoa beta)
  RB2W/1(Rw2b) -> RW2B/1

== system FixedWing_Dynamic_Model_SIL_simulink_PX4_H200/Dynamics/H200 Fixed-wing UAV Dynamics/Force and Moment Calculation/Aerodynamic Forces and Moments/Compute Body Frame Forces and Moments/Rotate FM to body frame/Rotate Moments ==
  alpha_beta : Inport
  M_w : Inport  Port=2
  Matrix Multiply : Product  Multiplication=Matrix(*)
  RB2W : Subsystem
  RW2B : Math  Operator=transpose  SignedPower=on
  M_b : Outport  PortDimensions=3  VectorParamsAs1DForOutWhenUnconnected=off
  wires:
  RB2W/1(Rw2b) -> RW2B/1
  alpha_beta/1 -> RB2W/1(aoa beta)
  M_w/1 -> Matrix Multiply/2
  RW2B/1 -> Matrix Multiply/1
  Matrix Multiply/1 -> M_b/1

== system FixedWing_Dynamic_Model_SIL_simulink_PX4_H200/Dynamics/H200 Fixed-wing UAV Dynamics/Force and Moment Calculation/Aerodynamic Forces and Moments/Compute Body Frame Forces and Moments/Wind frame F& M/Get Forces and Moments ==
  Airdata : Inport
  AeroCoeffs : Inport  Port=2
  Bus Selector : BusSelector  OutputSignals=signal2.CD,signal1.CY,signal2.CL
  Bus Selector3 : BusSelector  OutputSignals=signal1.Cl,signal1.Cn,signal2.Cm
  Bus Selector5 : BusSelector  OutputSignals=q
  Fx_a(Drag) : Product  Inputs=**  SaturateOnIntegerOverflow=on  OutDataTypeStr=Inherit: Same as first input
  Fy_a(Side) : Product  SaturateOnIntegerOverflow=on  OutDataTypeStr=Inherit: Same as first input
  Fz_a(Lift) : Product  SaturateOnIntegerOverflow=on  OutDataTypeStr=Inherit: Same as first input
  Mux : Mux  Inputs=6
  Mx_a : Product  Inputs=3  SaturateOnIntegerOverflow=on  OutDataTypeStr=Inherit: Same as first input
  My_a : Product  Inputs=3  SaturateOnIntegerOverflow=on  OutDataTypeStr=Inherit: Same as first input
  Mz_a : Product  Inputs=3  SaturateOnIntegerOverflow=on  OutDataTypeStr=Inherit: Same as first input
  Product1 : Product  SaturateOnIntegerOverflow=on  OutDataTypeStr=Inherit: Same as first input
  Signal Specification : SignalSpecification  Unit=m
  Signal Specification1 : SignalSpecification  Unit=m
  Signal Specification2 : SignalSpecification  Unit=m^2
  chord : Constant  Value=uavData.geometry.cw  VectorParams1D=off
      settings: AttributesFormatString=%<Value>
  span : Constant  Value=uavData.geometry.bw  VectorParams1D=off
      settings: AttributesFormatString=%<Value>
  span1 : Constant  Value=uavData.geometry.Sw  VectorParams1D=off
      settings: AttributesFormatString=%<Value>
  FM_w : Outport  VectorParamsAs1DForOutWhenUnconnected=off
  wires:
  Mx_a/1 -> Mux/4  "Mx_a"
  Bus Selector/2 -> Fy_a(Side)/1  "<CY>"
  Fx_a(Drag)/1 -> Mux/1  "Fx_a"
  Bus Selector/1 -> Fx_a(Drag)/1  "<CD>"
  AeroCoeffs/1 -> Bus Selector/1, Bus Selector3/1
  My_a/1 -> Mux/5  "My_a"
  Fz_a(Lift)/1 -> Mux/3  "Fz_a"
  Mz_a/1 -> Mux/6  "Mz_a"
  Airdata/1 -> Bus Selector5/1
  chord/1 -> Signal Specification/1
  span/1 -> Signal Specification1/1
  Fy_a(Side)/1 -> Mux/2  "Fy_a"
  Mux/1 -> FM_w/1
  Bus Selector3/2 -> Mz_a/1  "<Cn>"
  Bus Selector/3 -> Fz_a(Lift)/1  "<CL>"
  Product1/1 -> Fx_a(Drag)/2, Fy_a(Side)/2, Fz_a(Lift)/2, Mx_a/2, My_a/2, Mz_a/2  "qS"
  span1/1 -> Signal Specification2/1
  Bus Selector3/1 -> Mx_a/1  "<Cl>"
  Bus Selector5/1 -> Product1/1  "<q>"
  Signal Specification/1 -> My_a/3
  Signal Specification1/1 -> Mz_a/3, Mx_a/3
  Signal Specification2/1 -> Product1/2
  Bus Selector3/3 -> My_a/1  "<Cm>"

== system FixedWing_Dynamic_Model_SIL_simulink_PX4_H200/Dynamics/H200 Fixed-wing UAV Dynamics/Force and Moment Calculation/Aerodynamic Forces and Moments/Compute Body Frame Forces and Moments/Wind frame F& M/Lateral Channel ==
  beta : Inport
  p,q,r : Inport  Port=2
  Airspeed : Inport  Port=3
  dR : Inport  Port=4
  deltaA : Inport  Port=5
  Bus Creator : BusCreator  Inputs=3
  CY : Subsystem
  Cl : Subsystem
  Cn : Subsystem
  To Workspace : ToWorkspace  VariableName=beta  SaveFormat=Timeseries  SampleTime=-1
  Lateral : Outport  VectorParamsAs1DForOutWhenUnconnected=off
  wires:
  Cl/1(Cl) -> Bus Creator/2  "Cl"
  Cn/1(Cn) -> Bus Creator/3  "Cn"
  CY/1(CY) -> Bus Creator/1  "CY"
  Bus Creator/1 -> Lateral/1
  beta/1 -> To Workspace/1, Cn/1(beta), Cl/1(beta), CY/1(beta)
  p,q,r/1 -> Cn/2(p,q,r), Cl/2(p,q,r), CY/2(p,q,r)
  Airspeed/1 -> Cn/3(Airspeed), Cl/3(Airspeed), CY/3(Airspeed)
  dR/1 -> Cn/4(deltaR), Cl/4(deltaR), CY/4(deltaR)
  deltaA/1 -> Cn/5(deltaA), Cl/5(deltaA), CY/5(deltaA)

== system FixedWing_Dynamic_Model_SIL_simulink_PX4_H200/Dynamics/H200 Fixed-wing UAV Dynamics/Force and Moment Calculation/Aerodynamic Forces and Moments/Compute Body Frame Forces and Moments/Wind frame F& M/Longitudinal Channel ==
  alpha : Inport
  Airpseed : Inport  Port=2
  p,q,r : Inport  Port=3
  dE : Inport  Port=4
  dF : Inport  Port=5
  Bus Creator : BusCreator  Inputs=3
  CD : Subsystem
  CL : Subsystem
  Cm : Subsystem
  Transfer Fcn : TransferFcn  Numerator=[1 0]  Denominator=[0.1 1]
  Y-down : Gain  Gain=-1  SaturateOnIntegerOverflow=on  OutDataTypeStr=Inherit: Same as input  ParamDataTypeStr=Inherit: Same as input
      settings: AttributesFormatString=%<Gain>
  Y-down1 : Gain  Gain=-1  SaturateOnIntegerOverflow=on  OutDataTypeStr=Inherit: Same as input  ParamDataTypeStr=Inherit: Same as input
      settings: AttributesFormatString=%<Gain>
  Longitudinal : Outport  VectorParamsAs1DForOutWhenUnconnected=off
  wires:
  Transfer Fcn/1 -> CL/2(alpha_dot), Cm/2(alpha_dot)
  Airpseed/1 -> CL/4(Airspeed), Cm/4(Airpseed)
  p,q,r/1 -> CL/3(p,q,r), Cm/3(p,q,r)
  dF/1 -> CL/6(deltaF), Cm/6(deltaF)
  Bus Creator/1 -> Longitudinal/1
  Cm/1(Cm) -> Bus Creator/3  "Cm"
  CL/1(CL) -> Y-down/1, CD/1(CL)
  dE/1 -> Cm/5(deltaE), CL/5(deltaE)
  Y-down/1 -> Bus Creator/2  "CL"
  CD/1(CD) -> Y-down1/1
  alpha/1 -> CL/1(alpha), Cm/1(alpha), Transfer Fcn/1
  Y-down1/1 -> Bus Creator/1  "CD"

== system FixedWing_Dynamic_Model_SIL_simulink_PX4_H200/Dynamics/H200 Fixed-wing UAV Dynamics/Force and Moment Calculation/Motor Model/Engine Model/Power Model/CP Model ==
  J : Inport
  Constant : Constant  Value=uavData.engine.propellerModel.CPModel.pCP0
  Constant1 : Constant  Value=3
  Constant2 : Constant  Value=4
  Constant3 : Constant  Value=5
  Constant4 : Constant  Value=6
  Gain : Gain  Gain=uavData.engine.propellerModel.CPModel.pCP2
  Gain1 : Gain  Gain=uavData.engine.propellerModel.CPModel.pCP1
  Gain2 : Gain  Gain=uavData.engine.propellerModel.CPModel.pCP3
  Gain3 : Gain  Gain=uavData.engine.propellerModel.CPModel.pCP4
  Gain4 : Gain  Gain=uavData.engine.propellerModel.CPModel.pCP5
  Gain5 : Gain  Gain=uavData.engine.propellerModel.CPModel.pCP6
  Power{,1..3} (4 alike) : Math  Operator=pow
  Saturation : Saturate  UpperLimit=1  LowerLimit=0
  Square : Math  Operator=square
  Sum : Sum  Inputs=+++++++
  CP : Outport
  wires:
  J/1 -> Saturation/1
  Saturation/1 -> Gain1/1, Power3/1, Power2/1, Power1/1, Power/1, Square/1
  Square/1 -> Gain/1
  Sum/1 -> CP/1
  Constant1/1 -> Power/2
  Power/1 -> Gain2/1
  Power1/1 -> Gain3/1
  Constant2/1 -> Power1/2
  Constant3/1 -> Power2/2
  Power2/1 -> Gain4/1
  Power3/1 -> Gain5/1
  Constant4/1 -> Power3/2
  Constant/1 -> Sum/7
  Gain5/1 -> Sum/1
  Gain4/1 -> Sum/2
  Gain3/1 -> Sum/3
  Gain2/1 -> Sum/4
  Gain/1 -> Sum/5
  Gain1/1 -> Sum/6

== system FixedWing_Dynamic_Model_SIL_simulink_PX4_H200/Dynamics/H200 Fixed-wing UAV Dynamics/Force and Moment Calculation/Motor Model/Engine Model/Power Model/Calculate Rho ==
  Airspeed : Inport
  q : Inport  Port=2
  Divide : Product  Inputs=*/
  Gain : Gain  Gain=2
  Square : Math  Operator=square
  rho : Outport
  wires:
  q/1 -> Gain/1
  Airspeed/1 -> Square/1
  Gain/1 -> Divide/1
  Square/1 -> Divide/2
  Divide/1 -> rho/1

== system FixedWing_Dynamic_Model_SIL_simulink_PX4_H200/Dynamics/H200 Fixed-wing UAV Dynamics/Force and Moment Calculation/Motor Model/Engine Model/Power Model/J model ==
  n : Inport
  V : Inport  Port=2
  Constant : Constant  Value=0
  Divide : Product  Inputs=*/
  Switch : Switch  Criteria=u2 > Threshold  SaturateOnIntegerOverflow=off  InputSameDT=off
  uavData.engine.bladeDiameter : Gain  Gain=uavData.engine.bladeDiameter
  J : Outport
  wires:
  n/1 -> Switch/2, uavData.engine.bladeDiameter/1
  uavData.engine.bladeDiameter/1 -> Divide/2
  V/1 -> Divide/1
  Divide/1 -> Switch/1
  Switch/1 -> J/1
  Constant/1 -> Switch/3

== system FixedWing_Dynamic_Model_SIL_simulink_PX4_H200/Dynamics/H200 Fixed-wing UAV Dynamics/Force and Moment Calculation/Motor Model/Engine Model/Power Model/N [Hz] model ==
  deltaP : Inport
  Saturation : Saturate  UpperLimit=1  LowerLimit=0
  uavData.engine.propellerModel.RPMModel.pn1 : Gain  Gain=uavData.engine.propellerModel.RPMModel.pn1
  n : Outport
  wires:
  uavData.engine.propellerModel.RPMModel.pn1/1 -> n/1
  deltaP/1 -> Saturation/1
  Saturation/1 -> uavData.engine.propellerModel.RPMModel.pn1/1

== system FixedWing_Dynamic_Model_SIL_simulink_PX4_H200/Dynamics/H200 Fixed-wing UAV Dynamics/Force and Moment Calculation/Motor Model/Engine Model/Power Model/Power ==
  n : Inport
  CP : Inport  Port=2
  rho : Inport  Port=3
  Constant : Constant  Value=uavData.engine.bladeDiameter
  Constant1 : Constant  Value=5
  Constant2 : Constant  Value=3
  Power : Math  Operator=pow
  Power1 : Math  Operator=pow
  Product : Product  Inputs=4
  P : Outport
  wires:
  Constant/1 -> Power/1
  Constant1/1 -> Power/2
  n/1 -> Power1/1
  Power1/1 -> Product/1
  CP/1 -> Product/2
  rho/1 -> Product/3
  Power/1 -> Product/4
  Product/1 -> P/1
  Constant2/1 -> Power1/2

== system FixedWing_Dynamic_Model_SIL_simulink_PX4_H200/Dynamics/H200 Fixed-wing UAV Dynamics/Force and Moment Calculation/Motor Model/Engine Model/Thurst Model/CT Model ==
  J : Inport
  Constant : Constant  Value=uavData.engine.propellerModel.CTModel.pCT0
  Constant1 : Constant  Value=3
  Gain : Gain  Gain=uavData.engine.propellerModel.CTModel.pCT2
  Gain1 : Gain  Gain=uavData.engine.propellerModel.CTModel.pCT1
  Gain2 : Gain  Gain=uavData.engine.propellerModel.CTModel.pCT3
  Power : Math  Operator=pow
  Saturation : Saturate  UpperLimit=1  LowerLimit=0
  Square : Math  Operator=square
  Sum : Sum  Inputs=++++
  CT : Outport
  wires:
  J/1 -> Saturation/1
  Saturation/1 -> Power/1, Square/1, Gain1/1
  Square/1 -> Gain/1
  Sum/1 -> CT/1  "CT_Model"
  Constant1/1 -> Power/2
  Power/1 -> Gain2/1
  Gain2/1 -> Sum/1
  Gain1/1 -> Sum/3
  Gain/1 -> Sum/2
  Constant/1 -> Sum/4

== system FixedWing_Dynamic_Model_SIL_simulink_PX4_H200/Dynamics/H200 Fixed-wing UAV Dynamics/Force and Moment Calculation/Motor Model/Engine Model/Thurst Model/Calculate Rho ==
  Airspeed : Inport
  q : Inport  Port=2
  Divide : Product  Inputs=*/
  Gain : Gain  Gain=2
  Square : Math  Operator=square
  rho : Outport
  wires:
  q/1 -> Gain/1
  Airspeed/1 -> Square/1
  Gain/1 -> Divide/1
  Square/1 -> Divide/2
  Divide/1 -> rho/1

== system FixedWing_Dynamic_Model_SIL_simulink_PX4_H200/Dynamics/H200 Fixed-wing UAV Dynamics/Force and Moment Calculation/Motor Model/Engine Model/Thurst Model/J model ==
  n : Inport
  V : Inport  Port=2
  Constant : Constant  Value=0
  Divide : Product  Inputs=*/
  Switch : Switch  Criteria=u2 > Threshold  SaturateOnIntegerOverflow=off  InputSameDT=off
  uavData.engine.bladeDiameter : Gain  Gain=uavData.engine.bladeDiameter
  J : Outport
  wires:
  n/1 -> Switch/2, uavData.engine.bladeDiameter/1
  uavData.engine.bladeDiameter/1 -> Divide/2
  V/1 -> Divide/1
  Divide/1 -> Switch/1
  Switch/1 -> J/1
  Constant/1 -> Switch/3

== system FixedWing_Dynamic_Model_SIL_simulink_PX4_H200/Dynamics/H200 Fixed-wing UAV Dynamics/Force and Moment Calculation/Motor Model/Engine Model/Thurst Model/N [Hz] model ==
  deltaP : Inport
  " " : Gain  Gain=uavData.engine.propellerModel.RPMModel.pn1
  Saturation : Saturate  UpperLimit=1  LowerLimit=0
  n : Outport
  wires:
  " "/1 -> n/1
  deltaP/1 -> Saturation/1
  Saturation/1 -> " "/1

== system FixedWing_Dynamic_Model_SIL_simulink_PX4_H200/Dynamics/H200 Fixed-wing UAV Dynamics/Force and Moment Calculation/Motor Model/Engine Model/Thurst Model/Thrust Force ==
  n : Inport
  CT : Inport  Port=2
  rho : Inport  Port=3
  Constant : Constant  Value=uavData.engine.bladeDiameter
  Constant1 : Constant  Value=4
  Power : Math  Operator=pow
  Product : Product  Inputs=4
  Square : Math  Operator=square
  T : Outport
  wires:
  Constant/1 -> Power/1
  n/1 -> Square/1
  Square/1 -> Product/1
  CT/1 -> Product/2
  rho/1 -> Product/3
  Product/1 -> T/1
  Power/1 -> Product/4
  Constant1/1 -> Power/2

== system FixedWing_Dynamic_Model_SIL_simulink_PX4_H200/Dynamics/H200 Fixed-wing UAV Dynamics/Force and Moment Calculation/Aerodynamic Forces and Moments/Compute Body Frame Forces and Moments/Rotate FM to body frame/Rotate Forces/RB2W ==
  aoa beta : Inport
  11 : Fcn  Expr=u[3]*u[4]
  12 : Fcn  Expr=u[2]
  13 : Fcn  Expr=u[1]*u[4]
  21 : Fcn  Expr=-u[3]*u[2]
  22 : Fcn  Expr=u[4]
  23 : Fcn  Expr=-u[1]*u[2]
  31 : Fcn  Expr=-u[1]
  32 : Fcn  Expr=0
  33 : Fcn  Expr=u[3]
  Mux : Mux  Inputs=2
  Mux3 : Mux  Inputs=9
  Reshape 9x1->3x3 : Reshape  OutputDimensionality=Customize  OutputDimensions=[3,3]
  sincos : Trigonometry  Operator=sincos
  Rw2b : Outport  VectorParamsAs1DForOutWhenUnconnected=off
  wires:
  Mux/1 -> 11/1, 21/1, 31/1, 12/1, 22/1, 32/1, 13/1, 23/1, 33/1
  aoa beta/1 -> sincos/1
  sincos/2 -> Mux/2
  sincos/1 -> Mux/1
  33/1 -> Mux3/9
  23/1 -> Mux3/8
  13/1 -> Mux3/7
  32/1 -> Mux3/6
  22/1 -> Mux3/5
  12/1 -> Mux3/4
  31/1 -> Mux3/3
  21/1 -> Mux3/2
  11/1 -> Mux3/1
  Reshape 9x1->3x3/1 -> Rw2b/1
  Mux3/1 -> Reshape 9x1->3x3/1

== system FixedWing_Dynamic_Model_SIL_simulink_PX4_H200/Dynamics/H200 Fixed-wing UAV Dynamics/Force and Moment Calculation/Aerodynamic Forces and Moments/Compute Body Frame Forces and Moments/Rotate FM to body frame/Rotate Moments/RB2W ==
  aoa beta : Inport
  11 : Fcn  Expr=u[3]*u[4]
  12 : Fcn  Expr=u[2]
  13 : Fcn  Expr=u[1]*u[4]
  21 : Fcn  Expr=-u[3]*u[2]
  22 : Fcn  Expr=u[4]
  23 : Fcn  Expr=-u[1]*u[2]
  31 : Fcn  Expr=-u[1]
  32 : Fcn  Expr=0
  33 : Fcn  Expr=u[3]
  Mux : Mux  Inputs=2
  Mux3 : Mux  Inputs=9
  Reshape 9x1->3x3 : Reshape  OutputDimensionality=Customize  OutputDimensions=[3,3]
  sincos : Trigonometry  Operator=sincos
  Rw2b : Outport  VectorParamsAs1DForOutWhenUnconnected=off
  wires:
  Mux/1 -> 11/1, 21/1, 31/1, 12/1, 22/1, 32/1, 13/1, 23/1, 33/1
  aoa beta/1 -> sincos/1
  sincos/2 -> Mux/2
  sincos/1 -> Mux/1
  33/1 -> Mux3/9
  23/1 -> Mux3/8
  13/1 -> Mux3/7
  32/1 -> Mux3/6
  22/1 -> Mux3/5
  12/1 -> Mux3/4
  31/1 -> Mux3/3
  21/1 -> Mux3/2
  11/1 -> Mux3/1
  Reshape 9x1->3x3/1 -> Rw2b/1
  Mux3/1 -> Reshape 9x1->3x3/1

== system FixedWing_Dynamic_Model_SIL_simulink_PX4_H200/Dynamics/H200 Fixed-wing UAV Dynamics/Force and Moment Calculation/Aerodynamic Forces and Moments/Compute Body Frame Forces and Moments/Wind frame F& M/Lateral Channel/CY ==
  beta : Inport
  p,q,r : Inport  Port=2
  Airspeed : Inport  Port=3
  deltaR : Inport  Port=4
  deltaA : Inport  Port=5
  CYDr : Constant  Value=uavData.aero.CYdeltaR
      settings: AttributesFormatString=%<Value>
  CYDr1 : Constant  Value=uavData.aero.CYdeltaA
      settings: AttributesFormatString=%<Value>
  CYb : Constant  Value=uavData.aero.CYbeta
      settings: AttributesFormatString=%<Value>
  Product : Product  SaturateOnIntegerOverflow=on  OutDataTypeStr=Inherit: Same as first input
  Product1 : Product  SaturateOnIntegerOverflow=on  OutDataTypeStr=Inherit: Same as first input
  Product2 : Product  SaturateOnIntegerOverflow=on  OutDataTypeStr=Inherit: Same as first input
  Sum2 : Sum  Inputs=+++++  SaturateOnIntegerOverflow=on
  roll / yaw rate factors : Subsystem
  CY : Outport  VectorParamsAs1DForOutWhenUnconnected=off
  wires:
  deltaR/1 -> Product1/2
  CYDr/1 -> Product1/1
  Product/1 -> Sum2/1
  Sum2/1 -> CY/1
  beta/1 -> Product/2
  CYb/1 -> Product/1
  CYDr1/1 -> Product2/1
  deltaA/1 -> Product2/2
  Product2/1 -> Sum2/5
  Product1/1 -> Sum2/4
  roll / yaw rate factors/1(CYp) -> Sum2/2
  roll / yaw rate factors/2(CYr) -> Sum2/3
  p,q,r/1 -> roll / yaw rate factors/1(p,q,r)
  Airspeed/1 -> roll / yaw rate factors/2(Airspeed)

== system FixedWing_Dynamic_Model_SIL_simulink_PX4_H200/Dynamics/H200 Fixed-wing UAV Dynamics/Force and Moment Calculation/Aerodynamic Forces and Moments/Compute Body Frame Forces and Moments/Wind frame F& M/Lateral Channel/Cl ==
  beta : Inport
  p,q,r : Inport  Port=2
  Airspeed : Inport  Port=3
  deltaR : Inport  Port=4
  deltaA : Inport  Port=5
  CYDr : Constant  Value=uavData.aero.CldeltaR
      settings: AttributesFormatString=%<Value>
  CYDr1 : Constant  Value=uavData.aero.CldeltaA
      settings: AttributesFormatString=%<Value>
  Clb : Constant  Value=uavData.aero.Clbeta
      settings: AttributesFormatString=%<Value>
  Product2 : Product  SaturateOnIntegerOverflow=on  OutDataTypeStr=Inherit: Same as first input
  Product3 : Product  SaturateOnIntegerOverflow=on  OutDataTypeStr=Inherit: Same as first input
  Product4 : Product  SaturateOnIntegerOverflow=on  OutDataTypeStr=Inherit: Same as first input
  Sum : Sum  Inputs=+++++  SaturateOnIntegerOverflow=on
  roll factors : Subsystem
  Cl : Outport  VectorParamsAs1DForOutWhenUnconnected=off
  wires:
  Airspeed/1 -> roll factors/2(Airspeed)
  p,q,r/1 -> roll factors/1(p,q,r)
  Product4/1 -> Sum/1  "Clb"
  Sum/1 -> Cl/1
  beta/1 -> Product4/2
  Clb/1 -> Product4/1
  CYDr1/1 -> Product3/1
  deltaR/1 -> Product2/2
  deltaA/1 -> Product3/2
  Product2/1 -> Sum/4
  CYDr/1 -> Product2/1
  Product3/1 -> Sum/5
  roll factors/1(Clp) -> Sum/2
  roll factors/2(Clr) -> Sum/3

== system FixedWing_Dynamic_Model_SIL_simulink_PX4_H200/Dynamics/H200 Fixed-wing UAV Dynamics/Force and Moment Calculation/Aerodynamic Forces and Moments/Compute Body Frame Forces and Moments/Wind frame F& M/Lateral Channel/Cn ==
  beta : Inport
  p,q,r : Inport  Port=2
  Airspeed : Inport  Port=3
  deltaR : Inport  Port=4
  deltaA : Inport  Port=5
  CnDa : Constant  Value=uavData.aero.CndeltaA
      settings: AttributesFormatString=%<Value>
  CnDr : Constant  Value=uavData.aero.CndeltaR
      settings: AttributesFormatString=%<Value>
  Cnb : Constant  Value=uavData.aero.Cnbeta
      settings: AttributesFormatString=%<Value>
  Product2 : Product  SaturateOnIntegerOverflow=on  OutDataTypeStr=Inherit: Same as first input
  Product3 : Product  SaturateOnIntegerOverflow=on  OutDataTypeStr=Inherit: Same as first input
  Product4 : Product  SaturateOnIntegerOverflow=on  OutDataTypeStr=Inherit: Same as first input
  Sum : Sum  Inputs=+++++  SaturateOnIntegerOverflow=on
  roll / yaw rate factors : Subsystem
  Cn : Outport  VectorParamsAs1DForOutWhenUnconnected=off
  wires:
  Airspeed/1 -> roll / yaw rate factors/2(Airspeed)
  p,q,r/1 -> roll / yaw rate factors/1(p,q,r)
  Cnb/1 -> Product4/1
  beta/1 -> Product4/2
  Sum/1 -> Cn/1
  Product4/1 -> Sum/1
  roll / yaw rate factors/1(Cnp) -> Sum/2
  roll / yaw rate factors/2(Cnr) -> Sum/3
  deltaR/1 -> Product2/2
  CnDr/1 -> Product2/1
  CnDa/1 -> Product3/1
  deltaA/1 -> Product3/2
  Product2/1 -> Sum/4
  Product3/1 -> Sum/5
